simulink model "korangbuoc"  (R2018b)
settings: Solver=FixedStepAuto  StartTime=0.0  StopTime=10.0  FixedStep=0.001  RelTol=1e-3
settings Model: Creator=User  LastModifiedBy=User

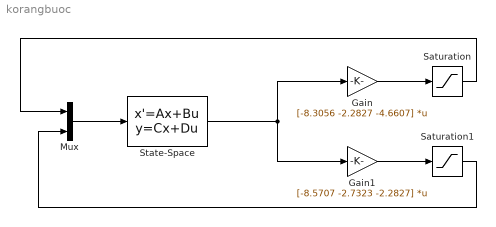
== system korangbuoc ==
  Gain : Gain  Gain=[-8.3056 -2.2827 -4.6607]  Multiplication=Matrix(K*u)
  Gain1 : Gain  Gain=[-8.5707 -2.7323 -2.2827]  Multiplication=Matrix(K*u)
  Mux : Mux  Inputs=2
  Saturation : Saturate  UpperLimit=3  LowerLimit=-3
  Saturation1 : Saturate  UpperLimit=20  LowerLimit=-20
  State-Space : StateSpace  A=[2 1 1;1 -1 0;0 0 1]  B=[0 0;0 1;1 0]  C=eye(3)  D=[0 0;0 0;0 0]  InitialCondition=[1;1;1]
  wires:
  State-Space/1 -> Gain/1, Gain1/1
  Gain/1 -> Saturation/1
  Gain1/1 -> Saturation1/1
  Mux/1 -> State-Space/1
  Saturation/1 -> Mux/1
  Saturation1/1 -> Mux/2
